simulink model "hyb_meas_dist_model"  (Simulink 5.0)
settings: Solver=ode45  StartTime=0.0  StopTime=Tstop  RelTol=1e-3
values from neighbouring files (symbols this model uses):
  HybMPC = hybcon(extended_plant,Q,N,limits,refs)    [hyb_integral_action.m]    (also in hyb_meas_dist.m)
libraries: hyblib x2, simulink x1
settings Model: LastModifiedBy=Alberto Bemporad  RTWOptions="-aEnforceIntegerDowncast=1 -aFoldNonRolledExpr=1 -aInlineInvariantSignals=0 -aInlineParameters=0 -aLocalBlockOutputs=1 -aRollThreshold=5 -aGenerateReport=0 -aGenCodeOnly=0 -aRTWVerbose=1 -aIncludeHyperlinkInReport=0 -aLaunchReport=0 -aForceParamTrailComments=0 -aGenerateComments=1 -aIgnoreCustomStorageClasses=1 -aIncHierarchyInIds=0 -aMaxRTWIdLen=31 -aShowEliminatedStatements=0 -aPrefixModelToSubsysFcnNames=1 -aIncDataTypeInIds=0 -aInsertBlockDesc=0 -aSimulinkBlockComments=1 -aInlinedPrmAccess=\"Literals\"  -aSuppressErrorStatus=0 -aModelReferenceCompliant=1 -aSupportNonInlinedSFcns=1 -aSupportContinuousTime=1 -aSupportComplex=1 -aSupportNonFinite=1 -aSupportAbsoluteTime=1 -aTargetPreCompLibLocation=\"\" -aTargetLibSuffix=\"\" -aTargetFcnLib=\"ansi_tfl_tmw.mat\" -aMultiInstanceERTCode=0 -aLogVarNameModifier=\"rt_\" -aIsPILTarget=0 -aCombineOutputUpdateFcns=0 -aGenerateASAP2=0 -aGenerateSampleERTMain=0 -aGenerateFullHeader=1 -aUtilityFuncGeneration=\"Auto\" -aIncludeFileDelimiter=\"Auto\" -aIncludeMdlTerminateFcn=1 -aPurelyIntegerCode=0 -aERTCustomFileBanners=0 -aRTWCAPIStates=0 -aRTWCAPIParams=0 -aRTWCAPISignals=0 -aMatFileLogging=1 -aGenFloatMathFcnCalls=\"ANSI_C\" -aExtModeMexFile=\"ext_comm\" -aExtModeTransport=0 -aExtModeStaticAllocSize=1000000 -aExtModeTesting=0 -aExtModeStaticAlloc=0 -aExtMode=0"

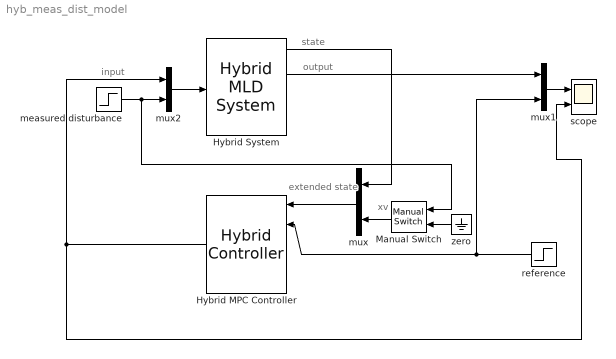
== system hyb_meas_dist_model ==
  note: state
  note: output
  note: input
  note: xv
  note: extended
      | state
  Hybrid MPC Controller : hyblib/Hybrid Controller  Orientation=left  C=HybMPC  S=extended_plant
  Hybrid System : hyblib/Hybrid MLD System  S=plant  x0init=x0
  Manual Switch : simulink/Signal Routing/Manual Switch  Orientation=left  sw=1  action=0
  measured disturbance : Step  Time=10  After=-0.5
  mux : Mux  Orientation=left  Inputs=2
  mux1 : Mux  Inputs=2
  mux2 : Mux  Inputs=2
  reference : Step  Orientation=left  Time=0  After=0.5
  scope : Scope  NumInputPorts=2
      settings: TimeRange=20  YMin=0~-1  YMax=1.5~0.5  DataFormat=Array  SampleTime=-1
  zero : Ground  Orientation=left
  wires:
  Hybrid System/2 -> mux1/1
  mux/1 -> Hybrid MPC Controller/1
  Hybrid System/1 -> mux/1
  mux1/1 -> scope/1
  reference/1 -> Hybrid MPC Controller/2, mux1/2
  mux2/1 -> Hybrid System/1
  Hybrid MPC Controller/1 -> mux2/1, scope/2
  measured disturbance/1 -> mux2/2, Manual Switch/1
  Manual Switch/1 -> mux/2
  zero/1 -> Manual Switch/2
